simulink model "simple_quarter_cjerk_ctrl_lqg"  (R2020b)
settings: Solver=ode15s  StartTime=0.0  StopTime=100  RelTol=1e-2
values from neighbouring files (symbols this model uses):
  estlqg = lqg(F,diag([1 0 0 1 0 10 1 .00001]),eye(11))    [quarter_jerk_ctrl.m]
  F = ss2ss(F,T)    [quarter_jerk_ctrl.m]
settings Model: Creator=Ricky  LastModifiedBy=Ricky

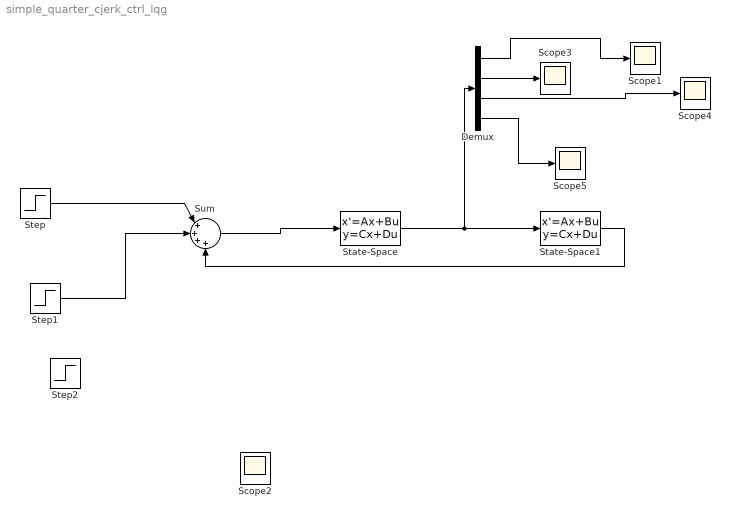
== system simple_quarter_cjerk_ctrl_lqg ==
  Demux : Demux
  Scope{1..5} (5 alike) : Scope
  State-Space : StateSpace  A=F.A  B=F.B  C=F.C  D=F.D  InitialCondition=0
  State-Space1 : StateSpace  A=estlqg.A  B=estlqg.B  C=estlqg.C  D=estlqg.D  InitialCondition=0
  Step : Step  SampleTime=0
  Step1 : Step  Time=2  After=-1  SampleTime=0
  Step2 : Step  Time=0  After=-1  SampleTime=0
  Sum : Sum  Inputs=|++++
  wires:
  Sum/1 -> State-Space/1
  Step/1 -> Sum/1
  Step1/1 -> Sum/2
  State-Space/1 -> Demux/1, State-Space1/1
  Demux/1 -> Scope1/1
  Demux/2 -> Scope3/1
  Demux/3 -> Scope4/1
  Demux/4 -> Scope5/1
  State-Space1/1 -> Sum/4
